simulink model "Antilock_Brake_System"  (R2020b)
settings: Solver=VariableStepAuto  StartTime=0.0  StopTime=10.0  RelTol=1e-3
values from neighbouring files (symbols this model uses):
  ctrl = 0    [ABS_Data.m]
  g = 32.18    [ABS_Data.m]
  I = 5    [ABS_Data.m]
  Kf = 1    [ABS_Data.m]
  m = 50    [ABS_Data.m]
  mu = [0 0.4 0.8 0.97 1.0 0.98 0.96 0.94 0.92 0.9 0.88 0.855 0.83 0.81 0.79 0.77 0.75 0.73 0.72 0.71 0.7]    [ABS_Data.m]
  PressureBrakemax = 1500    [ABS_Data.m]
  Rr = 15/12    (= 1.25)    [ABS_Data.m]
  slip = (0:0.05:1.0)    [ABS_Data.m]
  TB = 0.01    [ABS_Data.m]
  v0 = 88    [ABS_Data.m]
undefined symbols (not defined in the file or in its folder): sigbuilder_block
settings Model: Creator=vikas  LastModifiedBy=vikas

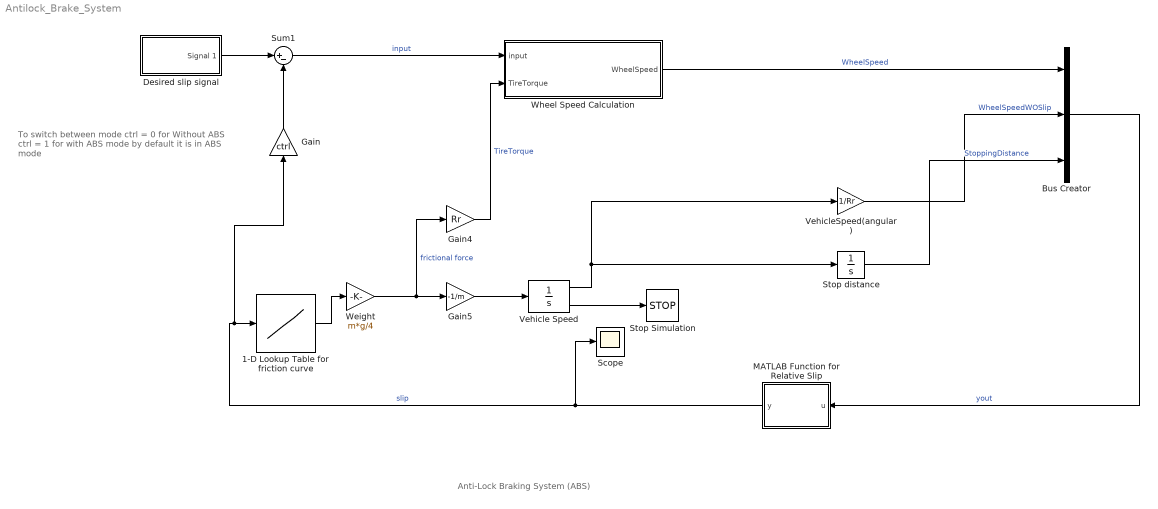
== system Antilock_Brake_System ==
  note: To switch between mode
      | ctrl = 0 for Without ABS
      | ctrl = 1 for with ABS mode
      | by default it is in ABS mode
  note: Anti-Lock Braking System (ABS)
  1-D Lookup Table for friction curve : Lookup_n-D  NumberOfTableDimensions=1  BreakpointsForDimension1=slip  Table=mu  InternalRulePriority=Speed  RndMeth=Simplest  InputSameDT=on
  Bus Creator : BusCreator  Inputs=3
  Desired slip signal : Subsystem  Tag=STV Subsys  LoadFcn=sigbuilder_block('load');  StartFcn=sigbuilder_block('start');  StopFcn=sigbuilder_block('stop');  ClipboardFcn=sigbuilder_block('clipboard');  mask(Sigbuilder block){tuvar=[0:10]}
      mask help: Simulink:masks:SigbuilderBlock_MD
      mask init:
      | if ~strcmp(get_param(bdroot(gcbh),'SimulationStatus'),'stopped') tuvar = sigbuilder_block('maskInit'); end
      settings: CopyFcn=sigbuilder_block('copy');  DeleteFcn=sigbuilder_block('delete');  ModelCloseFcn=sigbuilder_block('modelClose');  PreSaveFcn=sigbuilder_block('preSave');  PauseFcn=sigbuilder_block('pause');  ContinueFcn=sigbuilder_block('continue');  NameChangeFcn=sigbuilder_block('namechange');  OpenFcn=sigbuilder_block('open',[431.4 123 550.8 400.2 ]);  CloseFcn=sigbuilder_block('close');
      mask Display: plot(0, 0, 100, 100,[2, 2, 32, 32, 2], [68, 8, 8, 68, 68],[32, 2], [38, 38], [32, 19, 2],[53, 60, 44], [32, 17, 17, 2],[16, 16, 31, 31]);txt = getActiveGroup(gcbh);text(2, 100, txt,'verticalAlignment', 'top');
  Gain : Gain  Gain=ctrl
  Gain4 : Gain  Gain=Rr
  Gain5 : Gain  Gain=-1/m
  MATLAB Function for Relative Slip : MATLAB Function  TreatAsAtomicUnit=on
  Scope : Scope
  Stop Simulation : Stop
  Stop distance : Integrator
  Sum1 : Sum  Inputs=|+-
  Vehicle Speed : Integrator  InitialCondition=v0  LimitOutput=on  UpperSaturationLimit=1000  LowerSaturationLimit=0  ShowSaturationPort=on
  VehicleSpeed(angular) : Gain  Gain=1/Rr
  Weight : Gain  Gain=m*g/4
  Wheel Speed Calculation : Subsystem
  wires:
  Gain4/1 -> Wheel Speed Calculation/2(TireTorque)  "TireTorque"
  Desired slip signal/1(Signal 1) -> Sum1/1
  Wheel Speed Calculation/1(WheelSpeed) -> Bus Creator/1  "WheelSpeed"
  Sum1/1 -> Wheel Speed Calculation/1(input)  "input"
  Gain5/1 -> Vehicle Speed/1
  VehicleSpeed(angular)/1 -> Bus Creator/2  "WheelSpeedWOSlip"
  Bus Creator/1 -> MATLAB Function for Relative Slip/1(u)  "yout"
  Stop distance/1 -> Bus Creator/3  "StoppingDistance"
  Vehicle Speed/1 -> VehicleSpeed(angular)/1, Stop distance/1
  MATLAB Function for Relative Slip/1(y) -> Scope/1, Gain/1, 1-D Lookup Table for friction curve/1  "slip"
  Weight/1 -> Gain4/1, Gain5/1  "frictional force"
  1-D Lookup Table for friction curve/1 -> Weight/1
  Gain/1 -> Sum1/2
  Vehicle Speed/2 -> Stop Simulation/1

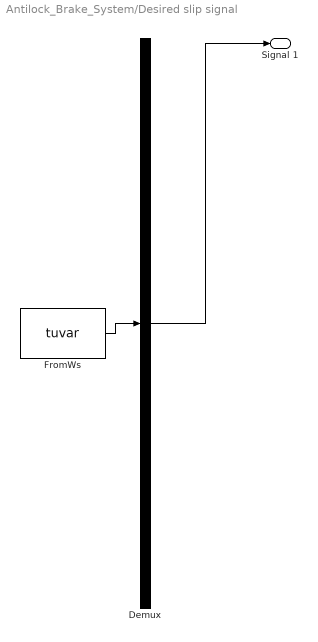
== system Antilock_Brake_System/Desired slip signal ==
  Demux : Demux  Tag=STV Demux  Outputs=1
      settings: DisplayOption=none
  FromWs : FromWorkspace  Tag=STV FromWs  VariableName=tuvar
      SigBuilderData=|
      | common.afterFinalStr = 'Extrapolate'
      | common.sampleTime = 0
      | dataSet.timeRange = [0 10]
      | dataSet.name = 'Group 1'
      | sbobj.Groups.Name = 'Group 1'
      | sbobj.Groups.Signals.Name = 'Signal 1'
      | sbobj.Groups.Signals.XData = [0 4 6 10]
      | sbobj.Groups.Signals.YData = [0.2 0.2 0.2 0.2]
  Signal 1 : Outport  Tag=STV Outport
  wires:
  Demux/1 -> Signal 1/1
  FromWs/1 -> Demux/1

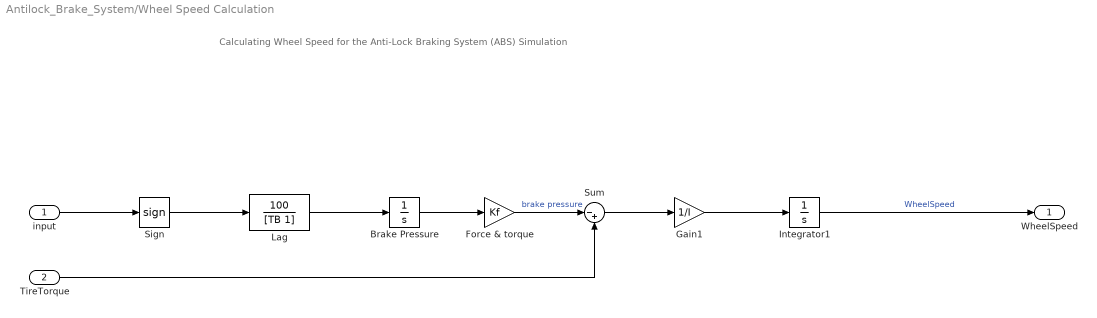
== system Antilock_Brake_System/Wheel Speed Calculation ==
  note: Calculating Wheel Speed for the Anti-Lock Braking System (ABS) Simulation
  input : Inport
  TireTorque : Inport  Port=2
  Brake Pressure : Integrator  LimitOutput=on  UpperSaturationLimit=PressureBrakemax  LowerSaturationLimit=0
  Force & torque : Gain  Gain=Kf
  Gain1 : Gain  Gain=1/I
  Integrator1 : Integrator  InitialCondition=v0/Rr  LimitOutput=on  UpperSaturationLimit=1000  LowerSaturationLimit=0
  Lag : TransferFcn  Numerator=[100]  Denominator=[TB 1]
  Sign : Signum
  Sum : Sum  Inputs=|-+
  WheelSpeed : Outport
  wires:
  Lag/1 -> Brake Pressure/1
  Sum/1 -> Gain1/1
  Sign/1 -> Lag/1
  Force & torque/1 -> Sum/1  "brake pressure"
  Brake Pressure/1 -> Force & torque/1
  Gain1/1 -> Integrator1/1
  TireTorque/1 -> Sum/2
  Integrator1/1 -> WheelSpeed/1  "WheelSpeed"
  input/1 -> Sign/1

== matlab function Antilock_Brake_System/MATLAB Function for Relative Slip ==
  data: u input; y output
function y = fcn(u)

y = 1.0-u(1)/(u(2) + (u(2)==0)*eps);
